simulink model "model_simple"  (R2019b)
settings: Solver=VariableStepAuto  StartTime=0.0  StopTime=10.0  RelTol=1e-3
values from neighbouring files (symbols this model uses):
  Cx = 1.15    [main.m]    (also in main_params_plot.m = 1.28)
  p_0 = -2.9998e-06    [main.m]    (also in main_params_plot.m = 1; measure.m = 1)
  p_1 = 0.32977    [main.m]    (also in main_params_plot.m = 1; measure.m = 1)
  p_2 = -0.0054782    [main.m]    (also in main_params_plot.m = 1; measure.m = 1)
  rho = 1.2    [main.m]    (also in main_params_plot.m)
settings Model: OrderedModelArguments=off  Creator=artof  LastModifiedBy=artof

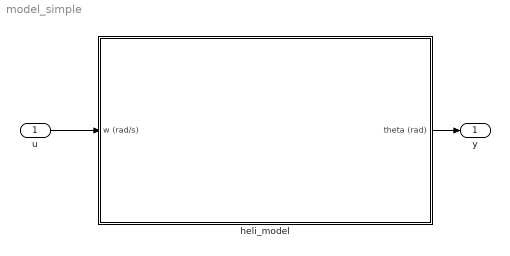
== system model_simple ==
  u : Inport
  heli_model : Subsystem
      mask Display: image('ident_model.png'); % Use "Edit Image" on toolstrip to change.
  "y " : Outport
  wires:
  u/1 -> heli_model/1(w (rad/s))
  heli_model/1(theta (rad)) -> "y "/1

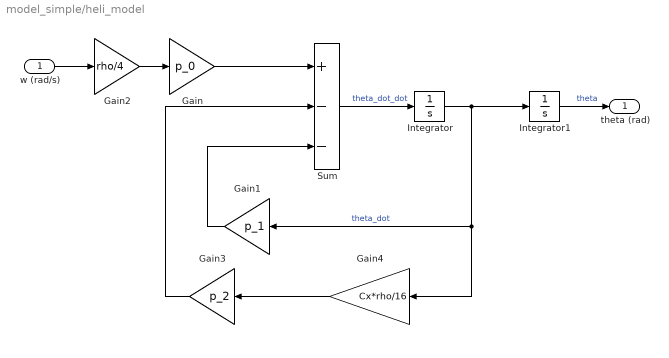
== system model_simple/heli_model ==
  w (rad/s) : Inport
  Gain : Gain  Gain=p_0
  Gain1 : Gain  Gain=p_1
  Gain2 : Gain  Gain=rho/4
  Gain3 : Gain  Gain=p_2
  Gain4 : Gain  Gain=Cx*rho/16
  Integrator : Integrator
  Integrator1 : Integrator
  Sum : Sum  Inputs=+--
  theta (rad) : Outport
  wires:
  Gain1/1 -> Sum/3
  Sum/1 -> Integrator/1  "theta_dot_dot"
  Gain/1 -> Sum/1
  Integrator/1 -> Integrator1/1, Gain4/1, Gain1/1  "theta_dot"
  Integrator1/1 -> theta (rad)/1  "theta"
  Gain3/1 -> Sum/2
  Gain2/1 -> Gain/1
  Gain4/1 -> Gain3/1
  w (rad/s)/1 -> Gain2/1
